simulink model "doc_scalar_quant_1"  (R2014a)
settings: Solver=ode45  StartTime=0.0  StopTime=12  RelTol=1e-3
libraries: simulink x1, commsrccod2 x1, dspsrcs4 x1
settings Model: Creator=The MathWorks Inc.
settings DataIOCC: SignalLoggingSaveFormat=ModelDataLogs  SignalLoggingName=logsOut
settings OptimizationCC: BlockReduction=off  BooleanDataType=off  ExpressionDepthLimit=2147483647
settings DebuggingCC: SaveWithParameterizedLinksMsg=none  UnderspecifiedInitializationDetection=Classic  SolverPrmCheckMsg=none  MultiTaskDSMMsg=warning  MultiTaskCondExecSysMsg=none  FcnCallInpInsideContextMsg=UseLocalSettings  StateNameClashWarn=warning  StrictBusMsg=None
settings HardwareCC: ProdHWDeviceType=Specified
settings RTWCC: IncludeERTFirstTime=on
settings CodeAppCC: MangleLength=5
settings GRTTargetCC: TargetFcnLib=iso_c_tmw.mat  CombineOutputUpdateFcns=off  GRTInterface=on

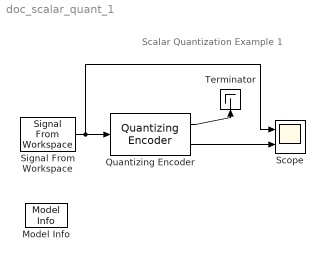
== system doc_scalar_quant_1 ==
  note: Scalar Quantization Example 1
  Model Info : simulink/Model-Wide Utilities/Model Info  InitialBlockCM=None  BlockCM=none  Frame=on  DisplayStringWithTags=Info  HorizontalTextAlignment=Center  LeftAlignmentValue=0.5  SourceBlockDiagram=doc_scalar_quant_1  TagMaxNumber=20
  Quantizing Encoder : commsrccod2/Quantizing Encoder  partition=[0,1,3]  codebook=[-1,.5,2,3]  idxDType=double
  Scope : Scope  NumInputPorts=2
      settings: YMin=-2.6~-2.6  YMax=3.7~3.7
  Signal From Workspace : dspsrcs4/Signal From Workspace  X=[-2.4, -1, -.2, 0, .2, 1, 1.2, 1.9, 2, 2.9, 3, 3.5]'  Ts=1  nsamps=1  OutputAfterFinalValue=Setting to zero  ignoreOrWarnInputAndFrameLengths=off
  Terminator : Terminator
  wires:
  Signal From Workspace/1 -> Scope/1, Quantizing Encoder/1
  Quantizing Encoder/1 -> Terminator/1
  Quantizing Encoder/2 -> Scope/2
